simulink model "drives"  (R2017b)
settings: Solver=VariableStepAuto  StartTime=0.0  StopTime=3  MaxStep=1e-4  RelTol=1e-3
libraries: powerlib x13, powerlib_meascontrol x2, simulink x1
settings Model: Creator=Ashish  LastModifiedBy=Ashish

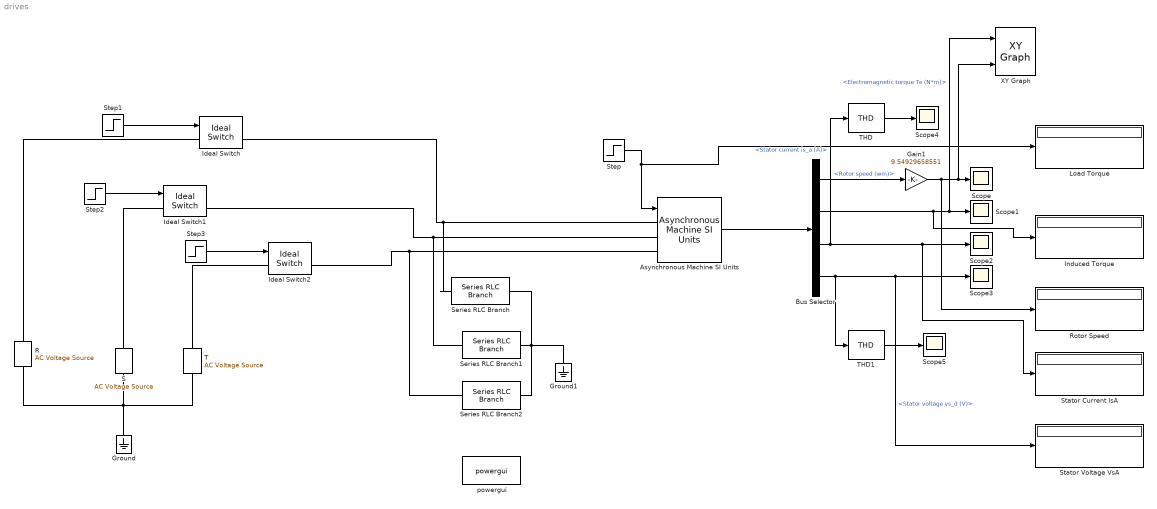
== system drives ==
  Asynchronous Machine SI Units : powerlib/Machines/Asynchronous Machine SI Units  RotorType=Squirrel-cage  PresetModel="15:  5.4 HP (4KW)   400 V  50Hz 1430 RPM"  MechanicalLoad=Torque Tm  ShowDetailedParameters=on  ReferenceFrame=Stationary  Units=SI  MeasurementBus=off  NominalParameters=[4000 400 50]  Stator=[1.405 0.005839]  Rotor=[1.395 0.005839]  Cage1=[0.4155 0.002066]  Cage2=[0.4168 0.0003495]  Lm=0.1722  Mechanical=[0.0131 0.002985 2]  PolePairs=2  InitialConditions=[0 0 0 0 0 0 0 0]  SimulateSaturation=off  Saturation=[14.03593122, 27.81365428, 53.79336849, 72.68890987, 97.98006896, 148.6815601, 215.7428561, 302.9841135, 428.7778367 ; 230, 322, 414, 460, 506, 552, 598, 644, 690]  LoadFlowParameters=1492000  TsPowergui=0  TsBlock=-1  IterativeModel=Trapezoidal non iterative  IterativeDiscreteModel=Trapezoidal non iterative  Pmec=1.492e+006
  Bus Selector : BusSelector  OutputSignals=Mechanical.Rotor speed (wm),Mechanical.Electromagnetic torque Te (N*m),Stator measurements.Stator current is_a (A),Stator measurements.Stator voltage vs_d (V)
  Gain1 : Gain  Gain=9.54929658551
  Ground : powerlib/Elements/Ground  LConnTagsString=a
  Ground1 : powerlib/Elements/Ground  LConnTagsString=a
  Ideal Switch : powerlib/Power Electronics/Ideal Switch  Ron=0.001  Lon=0  IC=0  Rs=1e5  Cs=inf  Measurements=on
  Ideal Switch1 : powerlib/Power Electronics/Ideal Switch  Ron=0.001  Lon=0  IC=0  Rs=1e5  Cs=inf  Measurements=on
  Ideal Switch2 : powerlib/Power Electronics/Ideal Switch  Ron=0.001  Lon=0  IC=0  Rs=1e5  Cs=inf  Measurements=on
  Induced Torque : Display
  Load Torque : Display
  R : powerlib/Electrical Sources/AC Voltage Source  Amplitude=325  Phase=0  Frequency=50  SampleTime=0  Measurements=None  BusType=swing  Pref=10e3  Qref=0  Qmin=-inf  Qmax=+inf
  Rotor Speed : Display
  S : powerlib/Electrical Sources/AC Voltage Source  Amplitude=325  Phase=-120  Frequency=50  SampleTime=0  Measurements=None  BusType=swing  Pref=10e3  Qref=0  Qmin=-inf  Qmax=+inf
  Scope{,1..5} (6 alike) : Scope
  Series RLC Branch : powerlib/Elements/Series RLC Branch  LConnTagsString=__new0  RConnTagsString=__new0  BranchType=RC  Resistance=10^-10  Inductance=10^-9  SetiL0=off  InitialCurrent=0  Capacitance=200*10^-6  Setx0=off  InitialVoltage=0  Measurements=None
  Series RLC Branch1 : powerlib/Elements/Series RLC Branch  LConnTagsString=__new0  RConnTagsString=__new0  BranchType=RC  Resistance=10^-10  Inductance=10^-9  SetiL0=off  InitialCurrent=0  Capacitance=200*10^-6  Setx0=off  InitialVoltage=0  Measurements=None
  Series RLC Branch2 : powerlib/Elements/Series RLC Branch  LConnTagsString=__new0  RConnTagsString=__new0  BranchType=RC  Resistance=10^-10  Inductance=10^-9  SetiL0=off  InitialCurrent=0  Capacitance=200*10^-6  Setx0=off  InitialVoltage=0  Measurements=None
  Stator Current IsA : Display
  "Stator Voltage VsA " : Display
  Step : Step  Time=0.5  Before=26.9  After=0  SampleTime=0
  Step1 : Step  Time=0.5  Before=1  After=0  SampleTime=0
  Step2 : Step  Time=0.5  Before=1  After=0  SampleTime=0
  Step3 : Step  Time=0.5  Before=1  After=0  SampleTime=0
  T : powerlib/Electrical Sources/AC Voltage Source  Amplitude=325  Phase=120  Frequency=50  SampleTime=0  Measurements=None  BusType=swing  Pref=10e3  Qref=0  Qmin=-inf  Qmax=+inf
  THD : powerlib_meascontrol/Measurements/THD  Freq=50  Ts=0
  THD1 : powerlib_meascontrol/Measurements/THD  Freq=50  Ts=0
  XY Graph : simulink/Sinks/XY Graph  xmin=-60  xmax=100  ymin=400  ymax=1650  st=0.001
  powergui : powerlib/powergui  Priority=1  SimulationMode=Continuous  SampleTime=50e-6  frequency=60  Iterations=50  frequencyindice=50  Pbase=100e6  ErrMax=1e-4  UnitsV=kV  UnitsW=MW  buscounter=0  FunctionMessages=off  echomessages=off  EnableUseOfTLC=off  CurrentSourceSwitches=off  DisableSnubberDevices=off  DisableRonSwitches=off  DisableVfSwitches=off  DisplayEquations=off  SolverType=Tustin/Backward Euler (TBE)  Interpol=off  ExternalGateDelay=off  methode=off  Ts=100  x0status=blocks  SPID=on  SwTol=0  HookPort=off  RestoreLinks=warning  ResistiveCurrentMeasurement=off  Frange=[0:2:500]  Ylog=off  Xlog=on  ShowGrid=off  save=off  variable=ZData  structure=0  ZoomFFT=off  StartTime=0.0  cycles=1  DisplayStyle=1  fundamental=60  FreqAxis=off  MaxFrequency=1000  frequencyindicesteady=1  RmsSteady=1  display=off
  wires:
  Asynchronous Machine SI Units/1 -> Bus Selector/1
  Bus Selector/3 -> THD/1, Stator Current IsA/1, Scope2/1  "<Stator current is_a (A)>"
  Bus Selector/2 -> Induced Torque/1, XY Graph/1, Scope1/1  "<Electromagnetic torque Te (N*m)>"
  Gain1/1 -> Rotor Speed/1, XY Graph/2, Scope/1
  Bus Selector/4 -> THD1/1, "Stator Voltage VsA "/1, Scope3/1  "<Stator voltage vs_d (V)>"
  THD/1 -> Scope4/1
  THD1/1 -> Scope5/1
  Bus Selector/1 -> Gain1/1  "<Rotor speed (wm)>"
  Step1/1 -> Ideal Switch/1
  Step2/1 -> Ideal Switch1/1
  Step3/1 -> Ideal Switch2/1
  Step/1 -> Load Torque/1, Asynchronous Machine SI Units/1
  connections:
  S/LConn1 -- T/LConn1 -- Ground/LConn1 -- R/LConn1
  Ideal Switch/RConn1 -- Series RLC Branch/LConn1 -- Asynchronous Machine SI Units/LConn1
  Ideal Switch1/RConn1 -- Series RLC Branch1/LConn1 -- Asynchronous Machine SI Units/LConn2
  Ideal Switch2/RConn1 -- Series RLC Branch2/LConn1 -- Asynchronous Machine SI Units/LConn3
  Series RLC Branch/RConn1 -- Ground1/LConn1 -- Series RLC Branch2/RConn1 -- Series RLC Branch1/RConn1
  Ideal Switch/LConn1 -- R/RConn1
  Ideal Switch1/LConn1 -- S/RConn1
  Ideal Switch2/LConn1 -- T/RConn1
